simulink model "auto"  (R2018b)
settings: Solver=FixedStepAuto  StartTime=0.0  StopTime=2410  FixedStep=sampletime  RelTol=1e-3
values from neighbouring files (symbols this model uses):
  Af = 2.34    [Auto_modell.m]    (also in Motor_modell.m)
  alfa = atan(slope/100)    [Auto_modell.m]    (also in Motor_modell.m)
  cd = 0.24    [Auto_modell.m]    (also in Motor_modell.m)
  fl = 0.88    [Auto_modell.m]    (also in Motor_modell.m)
  g = 9.81    [Auto_modell.m]    (also in Motor_modell.m)
  k = (0.5334/2)    (= 0.2667)    [Auto_modell.m]    (also in Motor_modell.m)
  m = 2108    [Auto_modell.m]    (also in Motor_modell.m)
  M = 300    [Auto_modell.m]    (also in Motor_modell.m)
  ro = 1.1846    [Auto_modell.m]    (also in Motor_modell.m)
  v = 150/3.6    (= 41.6666666667)    [Auto_modell.m]    (also in Motor_modell.m)
undefined symbols (not defined in the file or in its folder): input
settings Model: Creator=Lac  LastModifiedBy=Lac

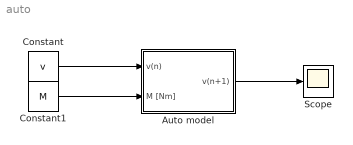
== system auto ==
  Auto model : Subsystem
  Constant : Constant  Value=v
  Constant1 : Constant  Value=M
  Scope : Scope
  wires:
  Constant/1 -> Auto model/1(v(n))
  Constant1/1 -> Auto model/2("M [Nm] ")
  Auto model/1(v(n+1)) -> Scope/1

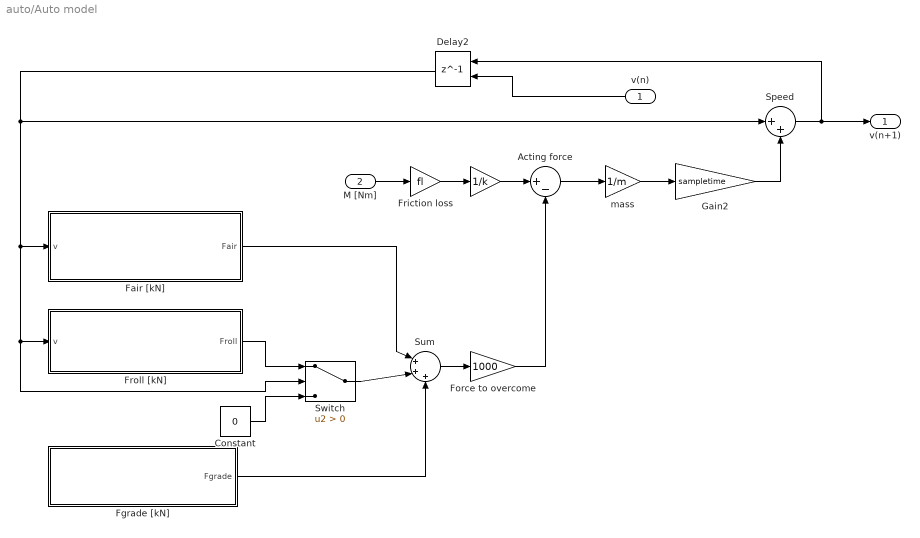
== system auto/Auto model ==
  v(n) : Inport
  "M [Nm] " : Inport  Port=2
  " " : Gain  Gain=1/k
  "Acting force " : Sum  Inputs=|+-
  Constant : Constant  Value=0
  Delay2 : Delay  DelayLength=1  InitialConditionSource=Input port  InitialCondition=input
      settings: InputPortMap=u0,p4
  "Fair [kN] " : Subsystem
  Fgrade [kN] : Subsystem
  Force to overcome : Gain  Gain=1000
  Friction loss : Gain  Gain=fl
  Froll [kN] : Subsystem
  Gain2 : Gain  Gain=sampletime
  "Speed " : Sum  Inputs=|++
  Sum : Sum  Inputs=|+++
  Switch : Switch  Criteria=u2 > Threshold
  mass : Gain  Gain=1/m
  v(n+1) : Outport
  wires:
  Delay2/1 -> Switch/2, Froll [kN]/1(v), "Fair [kN] "/1(v), "Speed "/1
  " "/1 -> "Acting force "/1
  Force to overcome/1 -> "Acting force "/2
  Constant/1 -> Switch/3
  Switch/1 -> Sum/2
  "Speed "/1 -> v(n+1)/1, Delay2/1
  mass/1 -> Gain2/1
  Sum/1 -> Force to overcome/1
  Gain2/1 -> "Speed "/2
  Fgrade [kN]/1(Fgrade) -> Sum/3
  "Fair [kN] "/1(Fair) -> Sum/1
  "Acting force "/1 -> mass/1
  v(n)/1 -> Delay2/2
  "M [Nm] "/1 -> Friction loss/1
  Friction loss/1 -> " "/1
  Froll [kN]/1(Froll) -> Switch/1

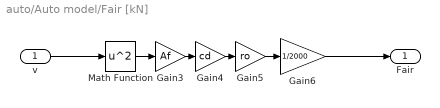
== system auto/Auto model/Fair [kN]  ==
  v : Inport
  Gain3 : Gain  Gain=Af
  Gain4 : Gain  Gain=cd
  Gain5 : Gain  Gain=ro
  Gain6 : Gain  Gain=1/2000
  Math Function : Math  Operator=square  SaturateOnIntegerOverflow=on
  Fair : Outport
  wires:
  Math Function/1 -> Gain3/1
  Gain4/1 -> Gain5/1
  Gain3/1 -> Gain4/1
  Gain5/1 -> Gain6/1
  v/1 -> Math Function/1
  Gain6/1 -> Fair/1

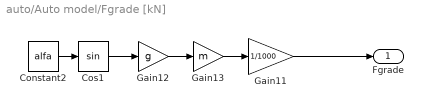
== system auto/Auto model/Fgrade [kN] ==
  Constant2 : Constant  Value=alfa
  Cos1 : Trigonometry
  Gain11 : Gain  Gain=1/1000
  Gain12 : Gain  Gain=g
  Gain13 : Gain  Gain=m
  Fgrade : Outport
  wires:
  Gain13/1 -> Gain11/1
  Constant2/1 -> Cos1/1
  Cos1/1 -> Gain12/1
  Gain12/1 -> Gain13/1
  Gain11/1 -> Fgrade/1

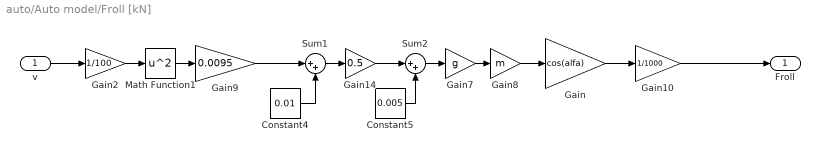
== system auto/Auto model/Froll [kN] ==
  v : Inport
  Constant4 : Constant  Value=0.01
  Constant5 : Constant  Value=0.005
  Gain : Gain  Gain=cos(alfa)
  Gain10 : Gain  Gain=1/1000
  Gain14 : Gain  Gain=0.5
  Gain2 : Gain  Gain=1/100
  Gain7 : Gain  Gain=g
  Gain8 : Gain  Gain=m
  Gain9 : Gain  Gain=0.0095
  Math Function1 : Math  Operator=square  SaturateOnIntegerOverflow=on
  Sum1 : Sum  Inputs=|++
  Sum2 : Sum  Inputs=|++
  Froll : Outport
  wires:
  Gain8/1 -> Gain/1
  Constant4/1 -> Sum1/2
  Sum2/1 -> Gain7/1
  Gain9/1 -> Sum1/1
  Sum1/1 -> Gain14/1
  Gain10/1 -> Froll/1
  Constant5/1 -> Sum2/2
  Math Function1/1 -> Gain9/1
  Gain14/1 -> Sum2/1
  Gain7/1 -> Gain8/1
  Gain2/1 -> Math Function1/1
  v/1 -> Gain2/1
  Gain/1 -> Gain10/1
